simulink model "Lab1_419_sim6"  (R2023b)
settings: Solver=VariableStepAuto  StartTime=0.0  StopTime=100  RelTol=1e-3
settings Model: Creator=julia  LastModifiedBy=julia

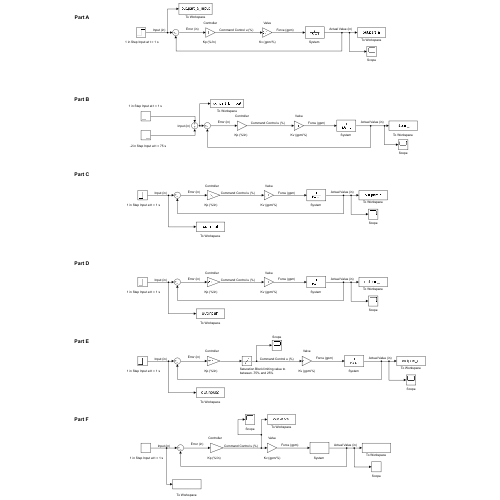
[thumbnail: Simulink's stored preview of the top-level diagram]
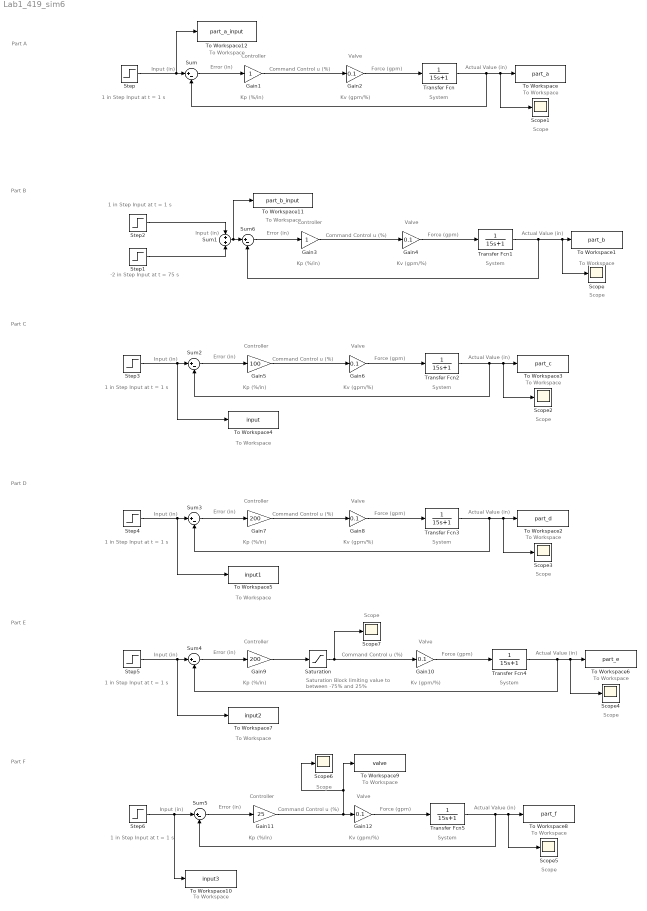
== system Lab1_419_sim6 ==
  note: System
  note: Saturation Block limiting value to between -75% and 25%
  note: Scope
  note: To Workspace
  note: Actual Value (in)
  note: Force (gpm)
  note: Controller
  note: Command Control u (%)
  note: Error (in)
  note: Kv (gpm/%)
  note: Valve
  note: Input (in)
  note: Kp (%/in)
  note: 1 in Step Input at t = 1 s
  note: Part A
  note: Part B
  note: Input (in)
  note: Force (gpm)
  note: Kv (gpm/%)
  note: Error (in)
  note: Actual Value (in)
  note: Kp (%/in)
  note: Controller
  note: Command Control u (%)
  note: Valve
  note: 1 in Step Input at t = 1 s
  note: -2 in Step Input at t = 75 s
  note: To Workspace
  note: Scope
  note: Input (in)
  note: To Workspace
  note: Force (gpm)
  note: Error (in)
  note: Kv (gpm/%)
  note: Valve
  note: To Workspace
  note: 1 in Step Input at t = 1 s
  note: Actual Value (in)
  note: Kp (%/in)
  note: Controller
  note: Command Control u (%)
  note: Scope
  note: Part C
  note: Input (in)
  note: Valve
  note: Kv (gpm/%)
  note: Error (in)
  note: To Workspace
  note: Force (gpm)
  note: Controller
  note: Part D
  note: Command Control u (%)
  note: Kp (%/in)
  note: Scope
  note: Actual Value (in)
  note: 1 in Step Input at t = 1 s
  note: To Workspace
  note: Kp (%/in)
  note: Scope
  note: Actual Value (in)
  note: Command Control u (%)
  note: 1 in Step Input at t = 1 s
  note: To Workspace
  note: Part E
  note: Controller
  note: Force (gpm)
  note: Input (in)
  note: Kv (gpm/%)
  note: Valve
  note: Error (in)
  note: To Workspace
  note: Kp (%/in)
  note: Scope
  note: Actual Value (in)
  note: Command Control u (%)
  note: 1 in Step Input at t = 1 s
  note: To Workspace
  note: Part F
  note: Controller
  note: Force (gpm)
  note: Input (in)
  note: Kv (gpm/%)
  note: Valve
  note: Error (in)
  note: To Workspace
  note: Scope
  note: To Workspace
  note: System
  note: System
  note: System
  note: System
  note: System
  note: Scope
  note: To Workspace
  note: To Workspace
  Gain1 : Gain
  Gain{2,4,6,8,10,12} (6 alike) : Gain  Gain=0.1
  Gain11 : Gain  Gain=25
  Gain3 : Gain
  Gain5 : Gain  Gain=100
  Gain7 : Gain  Gain=200
  Gain9 : Gain  Gain=200
  Saturation : Saturate  UpperLimit=25  LowerLimit=-75
  Scope{,1..7} (8 alike) : Scope
  Step{,2..6} (6 alike) : Step  SampleTime=1
  Step1 : Step  Time=75  Before=1  After=-1  SampleTime=1
  Sum{,2..6} (6 alike) : Sum  Inputs=|+-
  Sum1 : Sum
  To Workspace : ToWorkspace  VariableName=part_a  SampleTime=-1
  To Workspace1 : ToWorkspace  VariableName=part_b  SampleTime=-1
  To Workspace10 : ToWorkspace  VariableName=input3  SaveFormat=Timeseries  SampleTime=-1
  To Workspace11 : ToWorkspace  VariableName=part_b_input  SampleTime=-1
  To Workspace12 : ToWorkspace  VariableName=part_a_input  SampleTime=-1
  To Workspace2 : ToWorkspace  VariableName=part_d  SampleTime=-1
  To Workspace3 : ToWorkspace  VariableName=part_c  SampleTime=-1
  To Workspace4 : ToWorkspace  VariableName=input  SampleTime=-1
  To Workspace5 : ToWorkspace  VariableName=input1  SampleTime=-1
  To Workspace6 : ToWorkspace  VariableName=part_e  SampleTime=-1
  To Workspace7 : ToWorkspace  VariableName=input2  SampleTime=-1
  To Workspace8 : ToWorkspace  VariableName=part_f  SampleTime=-1
  To Workspace9 : ToWorkspace  VariableName=valve  SampleTime=-1
  Transfer Fcn{,1..5} (6 alike) : TransferFcn  Denominator=[15 1]
  wires:
  Step/1 -> To Workspace12/1, Sum/1
  Sum/1 -> Gain1/1
  Gain1/1 -> Gain2/1
  Gain2/1 -> Transfer Fcn/1
  Transfer Fcn/1 -> Sum/2, Scope1/1, To Workspace/1
  Sum1/1 -> To Workspace11/1, Sum6/1
  Transfer Fcn1/1 -> Scope/1, To Workspace1/1, Sum6/2
  Gain3/1 -> Gain4/1
  Gain4/1 -> Transfer Fcn1/1
  Step1/1 -> Sum1/2
  Step2/1 -> Sum1/1
  Gain5/1 -> Gain6/1
  Sum2/1 -> Gain5/1
  Transfer Fcn2/1 -> Sum2/2, Scope2/1, To Workspace3/1
  Step3/1 -> To Workspace4/1, Sum2/1
  Gain6/1 -> Transfer Fcn2/1
  Gain8/1 -> Transfer Fcn3/1
  Step4/1 -> To Workspace5/1, Sum3/1
  Sum3/1 -> Gain7/1
  Gain7/1 -> Gain8/1
  Transfer Fcn3/1 -> Sum3/2, Scope3/1, To Workspace2/1
  Transfer Fcn4/1 -> Sum4/2, Scope4/1, To Workspace6/1
  Step5/1 -> To Workspace7/1, Sum4/1
  Gain10/1 -> Transfer Fcn4/1
  Gain9/1 -> Saturation/1
  Sum4/1 -> Gain9/1
  Saturation/1 -> Scope7/1, Gain10/1
  Transfer Fcn5/1 -> Sum5/2, Scope5/1, To Workspace8/1
  Step6/1 -> To Workspace10/1, Sum5/1
  Gain12/1 -> Transfer Fcn5/1
  Gain11/1 -> Scope6/1, To Workspace9/1, Gain12/1
  Sum5/1 -> Gain11/1
  Sum6/1 -> Gain3/1
